simulink model "Project1"  (R2020a)
settings: Solver=VariableStepAuto  StartTime=0.0  StopTime=10.0  MaxStep=0.01  RelTol=1e-3
settings Model: Creator=cresp  LastModifiedBy=cresp

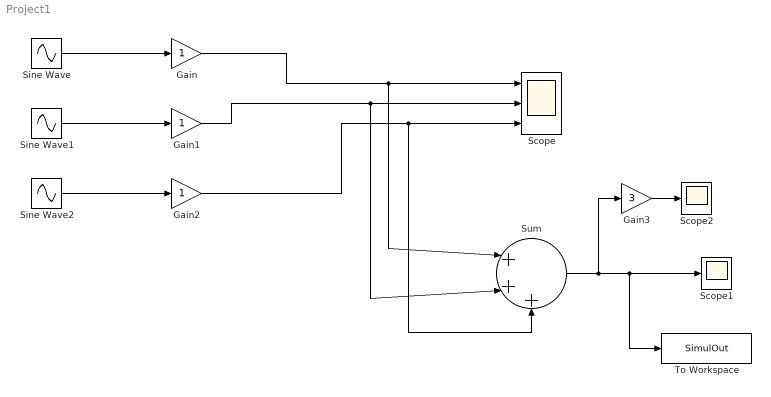
== system Project1 ==
  Gain : Gain
  Gain1 : Gain
  Gain2 : Gain
  Gain3 : Gain  Gain=3
  Scope : Scope  NumInputPorts=3
  Scope1 : Scope
  Scope2 : Scope
  Sine Wave : Sin  Frequency=2  SampleTime=0
  Sine Wave1 : Sin  Frequency=5  SampleTime=0
  Sine Wave2 : Sin  Frequency=10  SampleTime=0
  Sum : Sum  Inputs=|+++
  To Workspace : ToWorkspace  VariableName=SimulOut  SaveFormat=Timeseries  SampleTime=-1
  wires:
  Sine Wave/1 -> Gain/1
  Sine Wave1/1 -> Gain1/1
  Sine Wave2/1 -> Gain2/1
  Sum/1 -> Gain3/1, To Workspace/1, Scope1/1
  Gain/1 -> Sum/1, Scope/1
  Gain1/1 -> Sum/2, Scope/2
  Gain2/1 -> Sum/3, Scope/3
  Gain3/1 -> Scope2/1
